simulink model "Matlab"  (R2021b)
settings: Solver=VariableStepAuto  StartTime=0.0  StopTime=10.0  RelTol=1e-3
undefined symbols (not defined in the file or in its folder): A, B, C, Continuous, Time
libraries: ctrlSharedLib x1
settings Model: Creator=Reza Shahriari  LastModifiedBy=Reza Shahriari

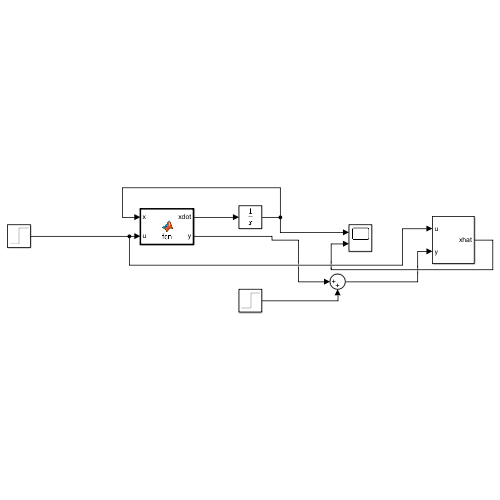
[thumbnail: Simulink's stored preview of the top-level diagram]
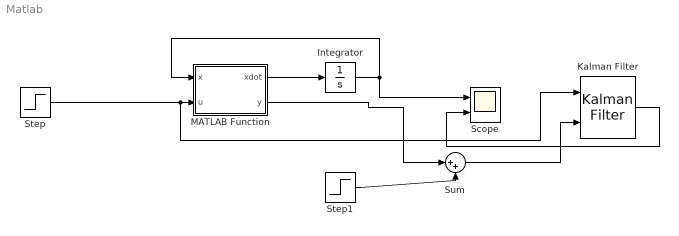
== system Matlab ==
  Integrator : Integrator  InitialCondition=[0;0]
  Kalman Filter : ctrlSharedLib/Kalman Filter  TimeDomain=Continuous-Time  UseCurrentEstimator=on  ModelSource=LTI State-Space Variable  ModelSourceVariable=ss(A,B,C,0,0)  A=0.95  B=1  C=1  D=0  NumberOfStates=1  NumberOfInputs=1  NumberOfOutputs=1  InitialEstimateSource=Dialog  X0=0  P0=10  UseK=off  UseGH=off  NumberOfProcessNoiseInputs=1  G=1  TimeInvariantG=on  H=0  TimeInvariantH=on  Q=0.05  TimeInvariantQ=on  R=1  TimeInvariantR=on  N=0  TimeInvariantN=on  AddInputPort=on  AddEnablePort=off  OutputEstimatedY=off  OutputP=off  Ts=-1
  MATLAB Function : MATLAB Function  TreatAsAtomicUnit=on
  Scope : Scope  NumInputPorts=2
  Step : Step  SampleTime=0
  Step1 : Step  SampleTime=0
  Sum : Sum  Inputs=|++
  wires:
  MATLAB Function/1(xdot) -> Integrator/1
  Integrator/1 -> Scope/1, MATLAB Function/1(x)
  Step/1 -> Kalman Filter/1, MATLAB Function/2(u)
  MATLAB Function/2(y) -> Sum/1
  Step1/1 -> Sum/2
  Sum/1 -> Kalman Filter/2
  Kalman Filter/1 -> Scope/2

== matlab function Matlab/MATLAB Function ==
  data: x input; xdot output; u input; y output
function [xdot , y]= fcn(x , u)

A = [-4.3340 -1.6200;1.0000 0]

B = [1;0]

C = [0 16.3300]
xdot = A*x + B*u
y = C*x
